simulink model "Simulator_Single_Axis"  (R2025a)
settings: Solver=ode45  StartTime=0.0  StopTime=simulation_time  RelTol=1e-6  AbsTol=1e-6
values from neighbouring files (symbols this model uses):
  A = [Xu, Xq, -9.81; Mu, Mq, 0; 0, 1, 0]    [Main_T1.m]
  B = [Xd; Md; 0]    [Main_T1.m]
  C = [1, 0, 0; 0, 1, 0; 0, 0, 1; Xu, Xq, 0]    [Main_T1.m]
  ctrl = parameters_controller()    [Main_T1.m]
  D = [0; 0; 0; Xd]    [Main_T1.m]
undefined symbols (not defined in the file or in its folder): delay, noise, seed
libraries: custom_PIDs_w_reset x2, simulink x1
settings Model: Creator=SalvatoreMeraglia  LastModifiedBy=lucaf
settings SolverCC: AlgebraicLoopSolver=TrustRegion
settings DebuggingCC: UnconnectedInputMsg=warning  UnconnectedOutputMsg=warning  UnconnectedLineMsg=warning
settings ModelReferenceCC: EnableRefExpFcnMdlSchedulingChecks=on
settings RTWCC: GPUComputeCapability=3.5  DLArmComputeVersion=19.05

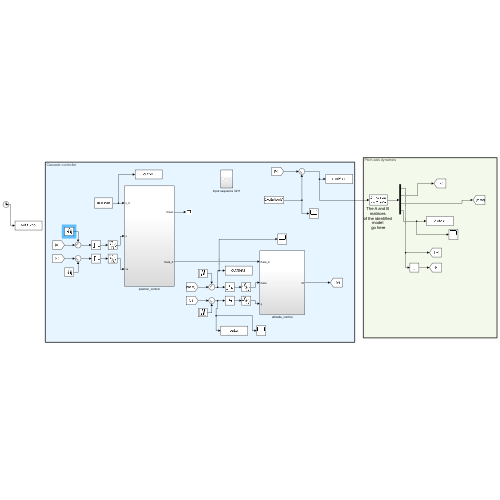
[thumbnail: Simulink's stored preview of the top-level diagram]
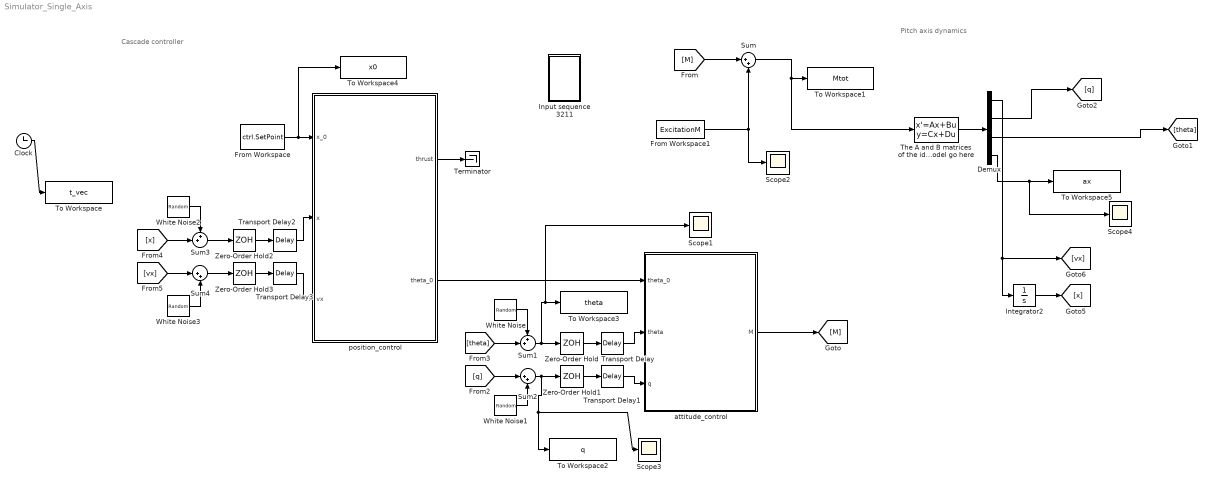
== system Simulator_Single_Axis ==
  note: Cascade controller
  note: Pitch axis dynamics
  Clock : Clock
  Demux : Demux
  From Workspace : FromWorkspace  VariableName=ctrl.SetPoint  SampleTime=ctrl.sample_time  OutputAfterFinalValue=Setting to zero
  From Workspace1 : FromWorkspace  VariableName=ExcitationM  SampleTime=ctrl.sample_time  OutputAfterFinalValue=Setting to zero
  Input sequence 3211 : Subsystem
  Integrator2 : Integrator
  Scope{1..4} (4 alike) : Scope
      Scope1 settings: ActiveDisplayYMinimum=-2.36747  ActiveDisplayYMaximum=2.35714
      Scope2 settings: ActiveDisplayYMinimum=-1  ActiveDisplayYMaximum=1
      Scope3 settings: ActiveDisplayYMinimum=-14.48365  ActiveDisplayYMaximum=14.03518
      Scope4 settings: ActiveDisplayYMinimum=-2.36747  ActiveDisplayYMaximum=2.35714
  Sum : Sum  Inputs=|++
  Sum1 : Sum  Inputs=++|
  Sum2 : Sum  Inputs=|++
  Sum3 : Sum  Inputs=++|
  Sum4 : Sum  Inputs=|++
  Terminator : Terminator
  The A and B matrices of the identified model go here : StateSpace  A=A  B=B  C=C  D=D  InitialCondition=0
  To Workspace : ToWorkspace  VariableName=t_vec  SampleTime=-1
  To Workspace1 : ToWorkspace  VariableName=Mtot  SampleTime=ctrl.sample_time
  To Workspace2 : ToWorkspace  VariableName=q  SampleTime=ctrl.sample_time
  To Workspace3 : ToWorkspace  VariableName=theta  SampleTime=ctrl.sample_time
  To Workspace4 : ToWorkspace  VariableName=x0  SampleTime=ctrl.sample_time
  To Workspace5 : ToWorkspace  VariableName=ax  SampleTime=ctrl.sample_time
  Transport Delay : TransportDelay  DelayTime=delay.attitude_filter * ctrl.sample_time
  Transport Delay1 : TransportDelay  DelayTime=delay.attitude_filter * ctrl.sample_time
  Transport Delay2 : TransportDelay  DelayTime=delay.position_filter * ctrl.sample_time
  Transport Delay3 : TransportDelay  DelayTime=delay.position_filter * ctrl.sample_time
  White Noise : RandomNumber  DisableCoverage=on  Variance=noise.attitude_stand_dev^2  Seed=seed.theta  SampleTime=ctrl.sample_time
  White Noise1 : RandomNumber  DisableCoverage=on  Variance=noise.ang_rate_stand_dev^2  Seed=seed.q  SampleTime=ctrl.sample_time
  White Noise2 : RandomNumber  DisableCoverage=on  Variance=noise.pos_stand_dev^2  Seed=seed.x  SampleTime=ctrl.sample_time
  White Noise3 : RandomNumber  DisableCoverage=on  Variance=noise.vel_stand_dev^2  Seed=seed.vx  SampleTime=ctrl.sample_time
  Zero-Order Hold{,1..3} (4 alike) : ZeroOrderHold  SampleTime=ctrl.sample_time
  attitude_control : Subsystem
  position_control : Subsystem
  wires:
  Transport Delay2/1 -> position_control/2(x)
  Transport Delay3/1 -> position_control/3(vx)
  attitude_control/1(M) -> [M]
  position_control/2(theta_0) -> attitude_control/1(theta_0)
  position_control/1(thrust) -> Terminator/1
  Demux/3 -> [theta]
  [M] -> Sum/1
  Sum/1 -> The A and B matrices of the identified model go here/1, To Workspace1/1
  From Workspace/1 -> To Workspace4/1, position_control/1(x_0)
  From Workspace1/1 -> Scope2/1, Sum/2
  Zero-Order Hold1/1 -> Transport Delay1/1
  White Noise2/1 -> Sum3/1
  [theta] -> Sum1/2
  White Noise/1 -> Sum1/1
  Zero-Order Hold/1 -> Transport Delay/1
  [vx] -> Sum4/1
  White Noise3/1 -> Sum4/2
  Sum3/1 -> Zero-Order Hold2/1
  [x] -> Sum3/2
  Zero-Order Hold2/1 -> Transport Delay2/1
  Sum2/1 -> Scope3/1, To Workspace2/1, Zero-Order Hold1/1
  [q] -> Sum2/1
  Zero-Order Hold3/1 -> Transport Delay3/1
  Sum4/1 -> Zero-Order Hold3/1
  Sum1/1 -> Scope1/1, To Workspace3/1, Zero-Order Hold/1
  White Noise1/1 -> Sum2/2
  Transport Delay1/1 -> attitude_control/3(q)
  Transport Delay/1 -> attitude_control/2(theta)
  The A and B matrices of the identified model go here/1 -> Demux/1
  Demux/2 -> [q]
  Demux/1 -> [vx], Integrator2/1
  Integrator2/1 -> [x]
  Demux/4 -> Scope4/1, To Workspace5/1
  Clock/1 -> To Workspace/1

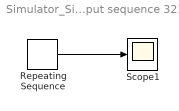
== system Simulator_Single_Axis/Input sequence 3211 ==
  Repeating Sequence : simulink/Sources/Repeating Sequence  rep_seq_t=[3 3.00001 5 5.00001 6 6.00001 7]  rep_seq_y=[1 -1 -1 1 1 -1 -1]
  Scope1 : Scope
      settings: ActiveDisplayYMinimum=-1  ActiveDisplayYMaximum=1.10549  DataLoggingVariableName=ScopeData2
  wires:
  Repeating Sequence/1 -> Scope1/1

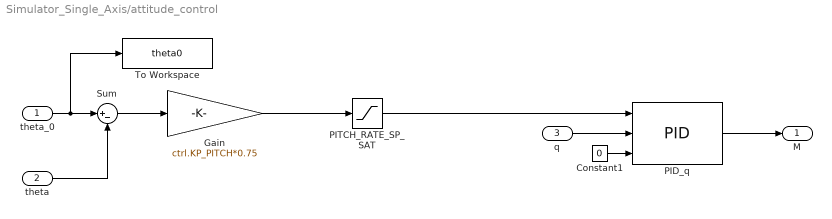
== system Simulator_Single_Axis/attitude_control ==
  theta_0 : Inport
  theta : Inport  Port=2
  q : Inport  Port=3
  Constant1 : Constant  Value=0  OutDataTypeStr=boolean
  Gain : Gain  Gain=ctrl.KP_PITCH*0.75
  PID_q : custom_PIDs_w_reset/PID  Kf=ctrl.KF_Q  Kp=ctrl.KP_Q  Ki=ctrl.KI_Q  Kd=ctrl.KD_Q  N=ctrl.N_filter_rate  min_u=ctrl.M_MIN  max_u=ctrl.M_MAX  ts=ctrl.sample_time
  PITCH_RATE_SP_SAT : Saturate  UpperLimit=ctrl.Q_MAX  LowerLimit=ctrl.Q_MIN
  Sum : Sum  Inputs=|+-
  To Workspace : ToWorkspace  VariableName=theta0  SampleTime=ctrl.sample_time
  M : Outport
  wires:
  PID_q/1 -> M/1
  q/1 -> PID_q/2
  PITCH_RATE_SP_SAT/1 -> PID_q/1
  Sum/1 -> Gain/1
  theta_0/1 -> To Workspace/1, Sum/1
  theta/1 -> Sum/2
  Gain/1 -> PITCH_RATE_SP_SAT/1
  Constant1/1 -> PID_q/3

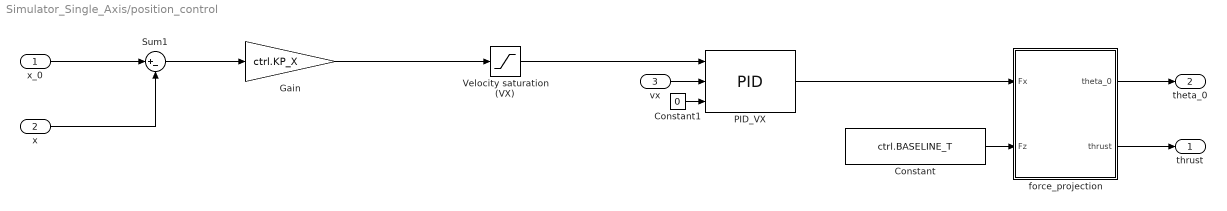
== system Simulator_Single_Axis/position_control ==
  x_0 : Inport
  x : Inport  Port=2
  vx : Inport  Port=3
  Constant : Constant  Value=ctrl.BASELINE_T
  Constant1 : Constant  Value=0  OutDataTypeStr=boolean
  Gain : Gain  Gain=ctrl.KP_X
  PID_VX : custom_PIDs_w_reset/PID  Kf=ctrl.KF_X_DOT  Kp=ctrl.KP_X_DOT  Ki=ctrl.KI_X_DOT  Kd=ctrl.KD_X_DOT  N=ctrl.N_filter_vel  min_u=ctrl.F_X_MIN  max_u=ctrl.F_X_MAX  ts=ctrl.sample_time
  Sum1 : Sum  Inputs=|+-
  Velocity saturation (VX) : Saturate  UpperLimit=ctrl.VEL_MAX  LowerLimit=ctrl.VEL_MIN
  force_projection : Subsystem
  thrust : Outport
  theta_0 : Outport  Port=2
  wires:
  vx/1 -> PID_VX/2
  Velocity saturation (VX)/1 -> PID_VX/1
  Sum1/1 -> Gain/1
  x_0/1 -> Sum1/1
  x/1 -> Sum1/2
  force_projection/2(thrust) -> thrust/1
  Gain/1 -> Velocity saturation (VX)/1
  Constant1/1 -> PID_VX/3
  Constant/1 -> force_projection/2(Fz)
  PID_VX/1 -> force_projection/1(Fx)
  force_projection/1(theta_0) -> theta_0/1

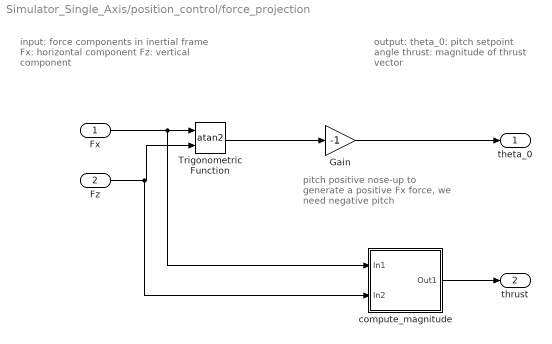
== system Simulator_Single_Axis/position_control/force_projection ==
  note: pitch positive nose-up
      | to generate a positive Fx force,
      | we need negative pitch
  note: output:
      | theta_0: pitch setpoint angle
      | thrust: magnitude of thrust vector
  note: input: force components in inertial frame
      | Fx: horizontal component
      | Fz: vertical component
  Fx : Inport
  Fz : Inport  Port=2
  Gain : Gain  Gain=-1
  Trigonometric Function : Trigonometry  Operator=atan2
  compute_magnitude : Subsystem
  theta_0 : Outport
  thrust : Outport  Port=2
  wires:
  Fx/1 -> compute_magnitude/1(In1), Trigonometric Function/1
  Fz/1 -> compute_magnitude/2(In2), Trigonometric Function/2
  Trigonometric Function/1 -> Gain/1
  Gain/1 -> theta_0/1
  compute_magnitude/1(Out1) -> thrust/1

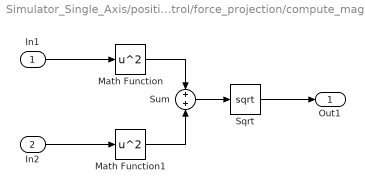
== system Simulator_Single_Axis/position_control/force_projection/compute_magnitude ==
  In1 : Inport
  In2 : Inport  Port=2
  Math Function : Math  Operator=square  SignedPower=on
  Math Function1 : Math  Operator=square  SignedPower=on
  Sqrt : Sqrt
  Sum : Sum
  Out1 : Outport
  wires:
  Sum/1 -> Sqrt/1
  Sqrt/1 -> Out1/1
  In1/1 -> Math Function/1
  Math Function1/1 -> Sum/2
  Math Function/1 -> Sum/1
  In2/1 -> Math Function1/1
